simulink model "Auto_microgrid_forecasting"  (R2020a)
settings: Solver=VariableStepAuto  StartTime=0.0  StopTime=40  MaxStep=1e-4  RelTol=1e-3
PreLoadFcn:
  | %load('GC_maxRPP_WS12_GHI790_BL330_nomSOC.mat')
InitFcn:
  | run('FC_microgrid_param.m')
  | tic
  | run('CARTinitFcn.m')
StopFcn:
  | toc
undefined symbols (not defined in the file or in its folder): breakpoints1, breakpoints2, cc_kp, cp_table_data, ctrl, D1, Delta, DiscIntNeverNeededParam, DT, FC_BESS, FC_PV_FirstSolar, find_system, Fnom, forecast, GC_mode, gcbh, GHI_rated, libFC_BESS, libFC_PV, LowerLimit, magnitude, oversize, pll_ki, pll_kp, Pmax_PV, Pmax_WT, sps_rtmsupport, timer, Ts, Ts_APC, Ts_Control, Ts_Power, U_rated, UpperLimit
libraries: powerlib x146, simulink x124, powerlib_extras x120, powerlib_meascontrol x94, eePowerMeasurement x28, pi_ctrl x20, simulink_extras x12, eeGeneralControl x10, sps_avr x7, libFSArray x2, libLgBattery x1, spsDieselMotorModel x1
(part 16 of 16)

== system Auto_microgrid_forecasting/MODEL STABILIZER/AllStringInverters/Stab_control/InvControl/PLL/PLL (3ph)1/Discrete ==
  note: Use internal or external tuning parameters
  Err : Inport  SampleTime=Ts
  Constant1 : Constant  Value=Kp
  Constant3 : Constant  Value=Ki
  Discrete-Time Integrator : DiscreteIntegrator  gainval=1  InitialCondition=Init  SampleTime=Ts  LimitOutput=on  UpperSaturationLimit=Par_Limits(1)  LowerSaturationLimit=Par_Limits(2)  ICPrevOutput=DiscIntNeverNeededParam  ICPrevScaledInput=DiscIntNeverNeededParam
  Product : Product
  Product1 : Product
  Saturation1 : Saturate  UpperLimit=Par_Limits(1)  LowerLimit=Par_Limits(2)  SampleTime=Ts
  Sum6 : Sum  InputSameDT=on  SaturateOnIntegerOverflow=on  SampleTime=Ts  OutDataTypeStr=Inherit: Same as first input
  Out : Outport  SampleTime=Ts  InitialOutput=0  VectorParamsAs1DForOutWhenUnconnected=off
  wires:
  Saturation1/1 -> Out/1
  Err/1 -> Product1/1, Product/2
  Sum6/1 -> Saturation1/1
  Product/1 -> Sum6/1
  Discrete-Time Integrator/1 -> Sum6/2
  Product1/1 -> Discrete-Time Integrator/1
  Constant1/1 -> Product/1  "Kp"
  Constant3/1 -> Product1/2  "Ki"

== system Auto_microgrid_forecasting/MODEL STABILIZER/AllStringInverters/Stab_control/InvControl/PLL/PLL (3ph)1/VCO ==
  w : Inport
  Compare To Constant : simulink/Logic and Bit Operations/Compare To Constant  relop=>=  const=pi  OutDataTypeStr=uint8
  Data Type Conversion : DataTypeConversion
  Gain : Gain  Gain=2*pi  OutDataTypeStr=double
  Gain2 : Gain  Gain=Ts  SaturateOnIntegerOverflow=on  OutDataTypeStr=Inherit: Same as input  ParamDataTypeStr=Inherit: Same as input
  Sum : Sum  Inputs=-++
  Unit Delay1 : UnitDelay  SampleTime=-1  HasFrameUpgradeWarning=on
  theta : Outport  VectorParamsAs1DForOutWhenUnconnected=off
  wires:
  w/1 -> Gain2/1
  Gain/1 -> Sum/1
  Compare To Constant/1 -> Data Type Conversion/1
  Unit Delay1/1 -> Compare To Constant/1, Sum/3, theta/1  "wt"
  Gain2/1 -> Sum/2
  Sum/1 -> Unit Delay1/1
  Data Type Conversion/1 -> Gain/1

== system Auto_microgrid_forecasting/Stab1/AllStringInverters/PV_Control/InvControl/PLL/PLL (3ph)1/Discrete ==
  note: Use internal or external tuning parameters
  Err : Inport  SampleTime=Ts
  Constant1 : Constant  Value=Kp
  Constant3 : Constant  Value=Ki
  Discrete-Time Integrator : DiscreteIntegrator  gainval=1  InitialCondition=Init  SampleTime=Ts  LimitOutput=on  UpperSaturationLimit=Par_Limits(1)  LowerSaturationLimit=Par_Limits(2)  ICPrevOutput=DiscIntNeverNeededParam  ICPrevScaledInput=DiscIntNeverNeededParam
  Product : Product
  Product1 : Product
  Saturation1 : Saturate  UpperLimit=Par_Limits(1)  LowerLimit=Par_Limits(2)  SampleTime=Ts
  Sum6 : Sum  InputSameDT=on  SaturateOnIntegerOverflow=on  SampleTime=Ts  OutDataTypeStr=Inherit: Same as first input
  Out : Outport  SampleTime=Ts  InitialOutput=0  VectorParamsAs1DForOutWhenUnconnected=off
  wires:
  Constant3/1 -> Product1/2  "Ki"
  Constant1/1 -> Product/1  "Kp"
  Product1/1 -> Discrete-Time Integrator/1
  Discrete-Time Integrator/1 -> Sum6/2
  Product/1 -> Sum6/1
  Sum6/1 -> Saturation1/1
  Err/1 -> Product/2, Product1/1
  Saturation1/1 -> Out/1

== system Auto_microgrid_forecasting/Stab1/AllStringInverters/PV_Control/InvControl/PLL/PLL (3ph)1/VCO ==
  w : Inport
  Compare To Constant : simulink/Logic and Bit Operations/Compare To Constant  relop=>=  const=pi  OutDataTypeStr=uint8
  Data Type Conversion : DataTypeConversion
  Gain : Gain  Gain=2*pi  OutDataTypeStr=double
  Gain2 : Gain  Gain=Ts  SaturateOnIntegerOverflow=on  OutDataTypeStr=Inherit: Same as input  ParamDataTypeStr=Inherit: Same as input
  Sum : Sum  Inputs=-++
  Unit Delay1 : UnitDelay  SampleTime=-1  HasFrameUpgradeWarning=on
  theta : Outport  VectorParamsAs1DForOutWhenUnconnected=off
  wires:
  Data Type Conversion/1 -> Gain/1
  Sum/1 -> Unit Delay1/1
  Gain2/1 -> Sum/2
  Unit Delay1/1 -> theta/1, Sum/3, Compare To Constant/1  "wt"
  Compare To Constant/1 -> Data Type Conversion/1
  Gain/1 -> Sum/1
  w/1 -> Gain2/1

== system Auto_microgrid_forecasting/Wind Turbine Type 4/Control/Measurement and Transformation/Discrete 3-phase PLL-Driven Positive-Sequence Active & Reactive Power/Discrete 3-phase PLL-Driven Positive-Sequence Fundamental Value/Discrete Variable Frequency Mean value1/Correction subsystem ==
  N : Inport
  F : Inport  Port=2
  In : Inport  Port=3
  Gain1 : Gain  Gain=0.5  SaturateOnIntegerOverflow=on  OutDataTypeStr=Inherit: Same as input  ParamDataTypeStr=Inherit: Same as input
  Product2 : Product  Inputs=*/  InputSameDT=on  SaturateOnIntegerOverflow=on  OutDataTypeStr=Inherit: Same as first input
  Product4 : Product  Inputs=**  InputSameDT=on  SaturateOnIntegerOverflow=on  OutDataTypeStr=Inherit: Same as first input
  Product5 : Product  Inputs=**  InputSameDT=on  SaturateOnIntegerOverflow=on  OutDataTypeStr=Inherit: Same as first input
  Sum1 : Sum  Inputs=+-  InputSameDT=on  SaturateOnIntegerOverflow=on  OutDataTypeStr=Inherit: Same as first input
  Sum4 : Sum  InputSameDT=on  SaturateOnIntegerOverflow=on  OutDataTypeStr=Inherit: Same as first input
  Sum5 : Sum  Inputs=+-  InputSameDT=on  SaturateOnIntegerOverflow=on  OutDataTypeStr=Inherit: Same as first input
  Unit Delay : UnitDelay  SampleTime=Ts  HasFrameUpgradeWarning=on
  Out : Outport  VectorParamsAs1DForOutWhenUnconnected=off
  wires:
  Product4/1 -> Out/1
  Sum4/1 -> Product4/2
  Gain1/1 -> Sum4/1
  Product5/1 -> Gain1/1
  Sum1/1 -> Product5/2
  In/1 -> Sum4/2, Unit Delay/1, Sum1/1
  Product2/1 -> Product4/1
  Sum5/1 -> Product5/1, Product2/1
  F/1 -> Sum5/2
  N/1 -> Product2/2, Sum5/1
  Unit Delay/1 -> Sum1/2

== system Auto_microgrid_forecasting/Wind Turbine Type 4/Control/Measurement and Transformation/Discrete 3-phase PLL-Driven Positive-Sequence Active & Reactive Power/Discrete 3-phase PLL-Driven Positive-Sequence Fundamental Value/Discrete Variable Frequency Mean value1/Discrete Variable Transport Delay ==
  In : Inport
  D : Inport  Port=2
  "S-Function " : S-Function  FunctionName=discreteVariableTransportDelay  Parameters=MaxDelay,Ts,InitialValue  SFunctionDeploymentMode=off  EnableBusSupport=off
  Out : Outport  VectorParamsAs1DForOutWhenUnconnected=off
  wires:
  D/1 -> "S-Function "/2
  In/1 -> "S-Function "/1
  "S-Function "/1 -> Out/1

== system Auto_microgrid_forecasting/Wind Turbine Type 4/Control/Measurement and Transformation/Discrete 3-phase PLL-Driven Positive-Sequence Active & Reactive Power/Discrete 3-phase PLL-Driven Positive-Sequence Fundamental Value/Discrete Variable Frequency Mean value2/Correction subsystem ==
  N : Inport
  F : Inport  Port=2
  In : Inport  Port=3
  Gain1 : Gain  Gain=0.5  SaturateOnIntegerOverflow=on  OutDataTypeStr=Inherit: Same as input  ParamDataTypeStr=Inherit: Same as input
  Product2 : Product  Inputs=*/  InputSameDT=on  SaturateOnIntegerOverflow=on  OutDataTypeStr=Inherit: Same as first input
  Product4 : Product  Inputs=**  InputSameDT=on  SaturateOnIntegerOverflow=on  OutDataTypeStr=Inherit: Same as first input
  Product5 : Product  Inputs=**  InputSameDT=on  SaturateOnIntegerOverflow=on  OutDataTypeStr=Inherit: Same as first input
  Sum1 : Sum  Inputs=+-  InputSameDT=on  SaturateOnIntegerOverflow=on  OutDataTypeStr=Inherit: Same as first input
  Sum4 : Sum  InputSameDT=on  SaturateOnIntegerOverflow=on  OutDataTypeStr=Inherit: Same as first input
  Sum5 : Sum  Inputs=+-  InputSameDT=on  SaturateOnIntegerOverflow=on  OutDataTypeStr=Inherit: Same as first input
  Unit Delay : UnitDelay  SampleTime=Ts  HasFrameUpgradeWarning=on
  Out : Outport  VectorParamsAs1DForOutWhenUnconnected=off
  wires:
  Unit Delay/1 -> Sum1/2
  N/1 -> Sum5/1, Product2/2
  F/1 -> Sum5/2
  Sum5/1 -> Product2/1, Product5/1
  Product2/1 -> Product4/1
  In/1 -> Sum1/1, Unit Delay/1, Sum4/2
  Sum1/1 -> Product5/2
  Product5/1 -> Gain1/1
  Gain1/1 -> Sum4/1
  Sum4/1 -> Product4/2
  Product4/1 -> Out/1

== system Auto_microgrid_forecasting/Wind Turbine Type 4/Control/Measurement and Transformation/Discrete 3-phase PLL-Driven Positive-Sequence Active & Reactive Power/Discrete 3-phase PLL-Driven Positive-Sequence Fundamental Value/Discrete Variable Frequency Mean value2/Discrete Variable Transport Delay ==
  In : Inport
  D : Inport  Port=2
  "S-Function " : S-Function  FunctionName=discreteVariableTransportDelay  Parameters=MaxDelay,Ts,InitialValue  SFunctionDeploymentMode=off  EnableBusSupport=off
  Out : Outport  VectorParamsAs1DForOutWhenUnconnected=off
  wires:
  "S-Function "/1 -> Out/1
  In/1 -> "S-Function "/1
  D/1 -> "S-Function "/2

== system Auto_microgrid_forecasting/Wind Turbine Type 4/Control/Measurement and Transformation/Discrete 3-phase PLL-Driven Positive-Sequence Active & Reactive Power/Discrete 3-phase PLL-Driven Positive-Sequence Fundamental Value2/Discrete Variable Frequency Mean value1/Correction subsystem ==
  N : Inport
  F : Inport  Port=2
  In : Inport  Port=3
  Gain1 : Gain  Gain=0.5  SaturateOnIntegerOverflow=on  OutDataTypeStr=Inherit: Same as input  ParamDataTypeStr=Inherit: Same as input
  Product2 : Product  Inputs=*/  InputSameDT=on  SaturateOnIntegerOverflow=on  OutDataTypeStr=Inherit: Same as first input
  Product4 : Product  Inputs=**  InputSameDT=on  SaturateOnIntegerOverflow=on  OutDataTypeStr=Inherit: Same as first input
  Product5 : Product  Inputs=**  InputSameDT=on  SaturateOnIntegerOverflow=on  OutDataTypeStr=Inherit: Same as first input
  Sum1 : Sum  Inputs=+-  InputSameDT=on  SaturateOnIntegerOverflow=on  OutDataTypeStr=Inherit: Same as first input
  Sum4 : Sum  InputSameDT=on  SaturateOnIntegerOverflow=on  OutDataTypeStr=Inherit: Same as first input
  Sum5 : Sum  Inputs=+-  InputSameDT=on  SaturateOnIntegerOverflow=on  OutDataTypeStr=Inherit: Same as first input
  Unit Delay : UnitDelay  SampleTime=Ts  HasFrameUpgradeWarning=on
  Out : Outport  VectorParamsAs1DForOutWhenUnconnected=off
  wires:
  Unit Delay/1 -> Sum1/2
  N/1 -> Sum5/1, Product2/2
  F/1 -> Sum5/2
  Sum5/1 -> Product2/1, Product5/1
  Product2/1 -> Product4/1
  In/1 -> Sum1/1, Unit Delay/1, Sum4/2
  Sum1/1 -> Product5/2
  Product5/1 -> Gain1/1
  Gain1/1 -> Sum4/1
  Sum4/1 -> Product4/2
  Product4/1 -> Out/1

== system Auto_microgrid_forecasting/Wind Turbine Type 4/Control/Measurement and Transformation/Discrete 3-phase PLL-Driven Positive-Sequence Active & Reactive Power/Discrete 3-phase PLL-Driven Positive-Sequence Fundamental Value2/Discrete Variable Frequency Mean value1/Discrete Variable Transport Delay ==
  In : Inport
  D : Inport  Port=2
  "S-Function " : S-Function  FunctionName=discreteVariableTransportDelay  Parameters=MaxDelay,Ts,InitialValue  SFunctionDeploymentMode=off  EnableBusSupport=off
  Out : Outport  VectorParamsAs1DForOutWhenUnconnected=off
  wires:
  "S-Function "/1 -> Out/1
  In/1 -> "S-Function "/1
  D/1 -> "S-Function "/2

== system Auto_microgrid_forecasting/Wind Turbine Type 4/Control/Measurement and Transformation/Discrete 3-phase PLL-Driven Positive-Sequence Active & Reactive Power/Discrete 3-phase PLL-Driven Positive-Sequence Fundamental Value2/Discrete Variable Frequency Mean value2/Correction subsystem ==
  N : Inport
  F : Inport  Port=2
  In : Inport  Port=3
  Gain1 : Gain  Gain=0.5  SaturateOnIntegerOverflow=on  OutDataTypeStr=Inherit: Same as input  ParamDataTypeStr=Inherit: Same as input
  Product2 : Product  Inputs=*/  InputSameDT=on  SaturateOnIntegerOverflow=on  OutDataTypeStr=Inherit: Same as first input
  Product4 : Product  Inputs=**  InputSameDT=on  SaturateOnIntegerOverflow=on  OutDataTypeStr=Inherit: Same as first input
  Product5 : Product  Inputs=**  InputSameDT=on  SaturateOnIntegerOverflow=on  OutDataTypeStr=Inherit: Same as first input
  Sum1 : Sum  Inputs=+-  InputSameDT=on  SaturateOnIntegerOverflow=on  OutDataTypeStr=Inherit: Same as first input
  Sum4 : Sum  InputSameDT=on  SaturateOnIntegerOverflow=on  OutDataTypeStr=Inherit: Same as first input
  Sum5 : Sum  Inputs=+-  InputSameDT=on  SaturateOnIntegerOverflow=on  OutDataTypeStr=Inherit: Same as first input
  Unit Delay : UnitDelay  SampleTime=Ts  HasFrameUpgradeWarning=on
  Out : Outport  VectorParamsAs1DForOutWhenUnconnected=off
  wires:
  Product4/1 -> Out/1
  Sum4/1 -> Product4/2
  Gain1/1 -> Sum4/1
  Product5/1 -> Gain1/1
  Sum1/1 -> Product5/2
  In/1 -> Sum4/2, Unit Delay/1, Sum1/1
  Product2/1 -> Product4/1
  Sum5/1 -> Product5/1, Product2/1
  F/1 -> Sum5/2
  N/1 -> Product2/2, Sum5/1
  Unit Delay/1 -> Sum1/2

== system Auto_microgrid_forecasting/Wind Turbine Type 4/Control/Measurement and Transformation/Discrete 3-phase PLL-Driven Positive-Sequence Active & Reactive Power/Discrete 3-phase PLL-Driven Positive-Sequence Fundamental Value2/Discrete Variable Frequency Mean value2/Discrete Variable Transport Delay ==
  In : Inport
  D : Inport  Port=2
  "S-Function " : S-Function  FunctionName=discreteVariableTransportDelay  Parameters=MaxDelay,Ts,InitialValue  SFunctionDeploymentMode=off  EnableBusSupport=off
  Out : Outport  VectorParamsAs1DForOutWhenUnconnected=off
  wires:
  D/1 -> "S-Function "/2
  In/1 -> "S-Function "/1
  "S-Function "/1 -> Out/1

== matlab function Auto_microgrid_forecasting/Wind Turbine Type 4/APC (atomic)1/Inertial Response (to df)1/FBIC/adaptive FBIC1 ==
  data: F_de input; Delta_P output; F_dr input; Wi input; P_de output; P_dr output; Act input
function [Delta_P,P_de,P_dr] = FBIC(F_de,F_dr,Wi,Act)
%Releasible kinetic energy based method by Dr. Kang 
if Act>=0.5
    
    Wmax=1;
    Wmin=0.9;
    R0=0.05;
    K0=1/R0/(Wmax^2-Wmin^2);
    
    Ri=R0*(Wmax^2-Wmin^2)/(Wi^2-Wmin^2);
    Ki=K0*(Wi^2-Wmin^2);
    P_dr=-1/Ri*F_dr;
    P_de=-Ki*F_de;
    Delta_P=P_dr+P_de;
else
    P_dr=0;
    P_de=0;
    Delta_P=0;
end

== matlab function Auto_microgrid_forecasting/Grid Feeder Protective Relay/R25 - Sync Check v0.1/deadbus fcn ==
  data: Vbus input; y output; Vline input
% Copyright (c) 2016 Massachusetts Institute of Technology
% Permission is hereby granted, free of charge, to any person obtaining a copy of this
% software and associated documentation files (the "Software"), to deal in the Software
% without restriction, including without limitation the rights to use, copy, modify,
% merge, publish, distribute, sublicense, and/or sell copies of the Software, and to
% permit persons to whom the Software is furnished to do so, subject to the following
% conditions:
%
%
% The above copyright notice and this permission notice shall be included in
% all copies or substantial portions of the Software.
%
% THE SOFTWARE IS PROVIDED "AS IS", WITHOUT WARRANTY OF ANY KIND, EXPRESS OR IMPLIED,
% INCLUDING BUT NOT LIMITED TO THE WARRANTIES OF MERCHANTABILITY, FITNESS FOR A
% PARTICULAR PURPOSE AND NONINFRINGEMENT. IN NO EVENT SHALL THE AUTHORS OR COPYRIGHT
% HOLDERS BE LIABLE FOR ANY CLAIM, DAMAGES OR OTHER LIABILITY, WHETHER IN AN ACTION
% OF CONTRACT, TORT OR OTHERWISE, ARISING FROM, OUT OF OR IN CONNECTION WITH THE
% SOFTWARE OR THE USE OR OTHER DEALINGS IN THE SOFTWARE.
%
%
%%

function y = fcn(Vbus, Vline)
%#codegen
if isnan(Vbus)
    Vbus=0;
elseif isnan(Vline)
    Vline = 0;
end

% voltage threshold for deadbus
threshold = 0.05; % @ 5%

% bounding open-circuit voltage at 120%
a = (Vbus>(0.8)) && (Vbus<1.20) && (Vline < threshold);
b = (Vline>(0.8)) && (Vline<1.20) && (Vbus < threshold);
c = (Vline<threshold) && (Vbus < threshold);
y = a||b||c;

== matlab function Auto_microgrid_forecasting/FC_PV_FirstSolar/MPPT Controller using Perturbe & Observe technique  ==
  settings: updateMethod=DISCRETE  sampleTime=Ts_Control
  data: Param input; Enabled input; V input; I input; D output
function D  = PandO(Param, Enabled, V, I)

% MPPT controller based on the Perturb & Observe algorithm.

% D output = Reference for DC link voltage (Vdc_ref) 
%
% Enabled input = 1 to enable the MPPT controller
% V input = PV array terminal voltage (V)
% I input = PV array current (A)
%
% Param input:
Dinit = Param(1);  %Initial value for Vdc_ref
Dmax = Param(2);   %Maximum value for Vdc_ref
Dmin = Param(3);   %Minimum value for Vdc_ref
deltaD = Param(4); %Increment value used to increase/decrease Vdc_ref
%  

persistent Vold Pold Dold;

dataType = 'double';

if isempty(Vold)
    Vold=0;
    Pold=0;
    Dold=Dinit;
end
P= V*I;
dV= V - Vold;
dP= P - Pold;

if dP ~= 0 & Enabled ~=0
    if dP < 0
        if dV < 0
            D = Dold + deltaD;
        else
            D = Dold - deltaD;
        end
    else
        if dV < 0
            D = Dold - deltaD;
        else
            D = Dold + deltaD;
        end    
    end
else D=Dold;
end

if D >= Dmax | D<= Dmin
    D=Dold;
end

Dold=D;
Vold=V;
Pold=P;

== matlab function Auto_microgrid_forecasting/Wind Turbine Type 4/Fault Controller (atomic) /turbine_safety  ==
  data: ctrl input Bus: ctrlBus; data input Bus: dataBus; ctrl output; timer input Bus: timerBus; timer output; faulty parameter; dt input
 function [ctrl, timer]   = turbine_safety(ctrl, data, timer, faulty, dt)
    % Fault adaptive controller. Checks various sensor readings, and
    % responds by entering the appropriate control mode, providing the
    % appropriate torque derate, and setting the appropriate timers.
          
    % if faulted, don't change anything 
    if ctrl.mode(4)+ctrl.mode(5)+ctrl.mode(6) == 0 %if not faulted
        ctrl.RP_prev = ctrl.mode(2); %0 if ctrl.cmd =0; 1 otherwise
        fields = fieldnames(faulty); %run warning logic for all faultys
        ctrl.mode = [0,0,0,0,0,0];
        for i=1:length(fields)
            ctrl.(fields{i}).state = 0;
            checkHandle = str2func(faulty.(fields{i}).checkFun); %check for warnings/faultys
            ctrl = checkHandle(data, ctrl);
            ctrl = setMode(ctrl, faulty, fields{i}); %set mode
        end
        [ctrl, timer] = setTimers(ctrl, timer, dt); %set timers and torque derate
        ctrl.modeValue = sum(ctrl.mode.*2.^linspace(0,5,6));
    else
        if ctrl.mode(6) == 1
            fprintf('EMERGENCY STOP')
        elseif ctrl.mode(5) == 1
            fprintf('OPEN LOOP NORMAL STOP')
        elseif ctrl.mode(4) == 1
            fprintf('NORMAL STOP')
        end

%     displays for testing
%         disp('ctrl.mode:')
%         disp(ctrl.mode)
%         disp('data:')
%         disp(data)
%         disp('timer:')
%         disp(timer)
%         fprintf('data = %1.0f\n', data);
%         fprintf('ctrl.Ttarget = %1.0f\n', ctrl.Ttarget);

    end

== matlab function Auto_microgrid_forecasting/Subsystem/MATLAB Function ==
  data: grid_disconnect output; f_B2 input; V_B2 input; f_B13 input; V_B13 input; PQ_CL input; PQ_NCL input; PQ_grid input; switch_grid input; PQ_BESS input; SOC_BESS input; PQ_WT input; switch_WT input; PQ_diesel input; switch_diesel input; PQ_PV input; Pest_WT input; Pest_PV input; grid_connect output; CL_switch output; NCL_switch output; BESS_switch output; BESS_mode output; BESS_PQ_cmd output; resync output; WT_switch_req output; WT_mode output; WT_PQ_cmd output; diesel_disconnect output; diesel_connect output; PV_switch output; PV_PQ_cmd output; PV_mode output; PQ_req input; timer input; timer output; try_island input; try_GC input; flag_hiSOC input; flag_hiSOC output; forecast parameter; targetSOC output; GC_mode parameter
function [grid_disconnect, grid_connect, CL_switch, NCL_switch, BESS_switch,...
    BESS_mode, BESS_PQ_cmd, resync, WT_switch_req,...
    WT_mode, WT_PQ_cmd, diesel_disconnect, diesel_connect, PV_switch,...
    PV_PQ_cmd, PV_mode, timer, flag_hiSOC, targetSOC] = fcn(f_B2, V_B2, f_B13, V_B13, PQ_CL, PQ_NCL, PQ_grid,...
    switch_grid, PQ_BESS, SOC_BESS, PQ_WT, switch_WT, PQ_diesel,...
    switch_diesel, PQ_PV, Pest_WT, Pest_PV, PQ_req, timer, try_island, try_GC, flag_hiSOC, forecast, GC_mode)
% Naming convention: for input signals, the asset comes last in the name.
% For output signals, the output comes first in the name

xloSOC = 0.01;
loSOC = 0.10;
hiSOC = 0.95;
xhiSOC = 0.99;
nomSOC = 0.7;
targetSOC = nomSOC;
SOCbuffer = 0.05;
% DEFAULT COMMANDS
WT_switch_req = 1;
PV_switch = 1;
diesel_connect = 0;
diesel_disconnect = 0;
grid_disconnect = 0;
grid_connect = 0;
CL_switch = 1;
NCL_switch = 1;
BESS_switch = 1;
BESS_mode = 1;
BESS_PQ_cmd = [1, 0];
resync = 0;
WT_mode = [2, 1]; % wind turbine modes [P_mode, Q_mode]. P_mode:1=inertial response, 2=primary frequency response, 3=cmd track, 4=MPPT. Q_mode: 1=voltage response, 2=momentary cessation, 3=cmd track, 4=zero.
WT_PQ_cmd = [1, 0];   % should I command this to balance power?
PV_PQ_cmd = [1, 0];  % should I command this to balance power?
BESS_PQ_cmd = [1, 0];
PV_mode = 0;  
P_WT = PQ_WT(1);
Q_WT = PQ_WT(2);
P_PV = PQ_PV(1);
Q_PV = PQ_PV(2);
Pmax_WT = 618460;
Qmax_WT = 618460;
Pmax_PV = 430000;
Qmax_PV = 430000;
Pmax_BESS = 1e6;
Pmin_BESS = -Pmax_BESS;
Qmax_BESS = 1e6;
Qmin_BESS = -Qmax_BESS;
U_rated = 12;  % m/s
U_min = 6;  % m/s
GHI_rated = 1000;  %W/m2

Pmin_WT = U_min^3/U_rated^3*Pmax_WT;
PQ_L = PQ_CL + PQ_NCL;
P_L = PQ_L(1);
Q_L = PQ_L(2);

f_grid_connect = 0.5; % Hz
V_grid_connect = 0.1; % pu
f_grid_discon = 1.8; % Hz
V_grid_discon = 0.3; % pu

if try_island == 0
    timer = 0;
end

switch switch_grid
    % ISLANDED CASE
    case 0
        targetSOC = targetSOC_from_forecast(forecast, U_rated, GHI_rated, Pmax_WT, Pmax_PV, U_min, nomSOC);
        WT_mode = [2, 1];
        try_island = 0; %time until islanded
        % CHOOSE BESS MODE BASED ON SOC
        if SOC_BESS > xhiSOC || SOC_BESS < xloSOC || BESS_switch == 0  % THINK ABOUT THIS LOGIC
            BESS_mode = 0; %GFL
            if switch_diesel == 0
                diesel_connect = 1;
            else
                 if SOC_BESS > xhiSOC
                    BESS_PQ_cmd = [-1, 0];
                 elseif SOC_BESS < xloSOC
                    BESS_PQ_cmd = [1, 0];
                 end
            end
        else
            BESS_mode = 1; %GFM
        end
    % CHOOSE MICROSOURCE DISPATCH BASED ON LOAD AND RESOURCE (LATER ADD
    % FORECASTING) % I think some quantities may need to be filtered or
    % time-averaged to prevent excessive switching around threshold levels
    if BESS_switch
        if P_L > (Pest_WT+ Pest_PV + Pmax_BESS) % connect diesel if other assets can't cover load
            if switch_diesel == 0
                diesel_connect = 1;
            end
        end
        if SOC_BESS < loSOC    
            if P_L > 0.9*(Pest_WT+ Pest_PV) % min(Pest_WT, P_wind)?
                disp('hi load')
                WT_switch_req = 1;
                PV_switch = 1;
                if switch_diesel == 0
                    diesel_connect = 1;
                    disp('diesel connect')
                end
        %     elseif P_L > 0.9*(Pest_WT)  
        %         WT_switch = 1;
        %         PV_switch = 1;
            else
                WT_switch_req = 1;  
                PV_switch = 1;
            end
        else
            if SOC_BESS < targetSOC
                PV_PQ_cmd =[10*(targetSOC-SOC_BESS), PV_PQ_cmd(2)];
            else
                PV_PQ_cmd = [((P_L - P_WT)/Pmax_PV), PV_PQ_cmd(2)]; % provide difference between load and wind turbine power with PV if not in loSOC
            end
        end
        
        if SOC_BESS > hiSOC
                diesel_disconnect = 1;
                PV_switch = 0;
                WT_switch_req = 0;
                flag_hiSOC = 1;
        elseif SOC_BESS > targetSOC && flag_hiSOC == 1
                PV_switch = 0;
                WT_switch_req = 0;
        elseif SOC_BESS > 0.4
            flag_hiSOC = 0;
            if P_L < (Pest_WT + Pest_PV + Pmax_BESS) && switch_diesel == 1
                diesel_disconnect = 1;
            end        
%                 if P_L < Pest_WT
%                     PV_switch = 0;
%                     WT_switch_req = 0;
%                 elseif P_L < (Pest_WT + Pest_PV)
%                     PV_switch = 0;
%                     WT_switch_req = 1;
%                 else
%                     PV_switch = 1;
%                     WT_switch_req = 1;
%                 end
        end
    end
    if try_GC % try to connect to the utility grid 
        if abs(f_B2-60) <= f_grid_connect && abs(V_B2-1) <= V_grid_connect % connect if grid stable enough
            resync = 1;
            grid_connect = 1;
        end
    end
        
        
    
    % GRID CONNECTED CASE
    case 1
        try_GC = 0;
        CL_switch = 1;
        NCL_switch = 1;
        if switch_diesel == 1
            diesel_disconnect = 1;
        end 
        hiSOC_droop = (SOC_BESS - (hiSOC - SOCbuffer))*10;
        loSOC_droop = -((loSOC + SOCbuffer) - SOC_BESS)*10;
        switch GC_mode
            case 1 % max renewable power production
                WT_switch_req = 1;
                PV_switch = 1;
                BESS_mode = 0;
                BESS_PQ_cmd = [10*(SOC_BESS-targetSOC) , 0]; % charge battery to SOC target
                WT_mode = [4, 4]; % check that my modes are updated everywhere.
                PV_PQ_cmd = [1, 0];
%                 if f_B13 > 60
%                     if SOC_BESS > (hiSOC - SOCbuffer) % if approaching hi state of charge, BESS will discharge
%                         BESS_mode = 0;
%                         BESS_PQ_cmd = [hiSOC_droop,  BESS_PQ_cmd(2)];%[max(BESS_PQ_cmd(1), 0), BESS_PQ_cmd(2)];
%                     else % if not, provide V/f droop support
%                         BESS_mode = 1;
%                     end
%                 elseif f_B13 < 60
%                     if SOC_BESS < (loSOC + SOCbuffer) % if approaching low state of charge, BESS will charge
%                         BESS_mode = 0;
%                         BESS_PQ_cmd = [loSOC_droop,  BESS_PQ_cmd(2)];%[min(BESS_PQ_cmd(1), 0), BESS_PQ_cmd(2)];
%                     else % if not, provide V/f droop support
%                         BESS_mode = 1;
%                     end
%                 end
            case 2 %grid support with V/f droop control
                WT_switch_req = 1;
                PV_switch = 1;
                WT_mode = [2, 1];
                PV_mode = 0;
                PV_PQ_cmd = [1, 0];
                BESS_mode = 0;
                BESS_PQ_cmd = [10*(SOC_BESS-targetSOC) , 0]; % charge battery to SOC target          
%                 if f_B13 > 60
%                     if SOC_BESS > (hiSOC - SOCbuffer) % if approaching hi state of charge, BESS will discharge
%                         BESS_mode = 0;
%                         BESS_PQ_cmd = [hiSOC_droop,  BESS_PQ_cmd(2)];%[max(BESS_PQ_cmd(1), 0), BESS_PQ_cmd(2)];
%                     else % if not, provide V/f droop support
%                         BESS_mode = 1;
%                     end
%                 elseif f_B13 < 60
%                     if SOC_BESS < (loSOC + SOCbuffer) % if approaching low state of charge, BESS will charge
%                         BESS_mode = 0;
%                         BESS_PQ_cmd = [loSOC_droop,  BESS_PQ_cmd(2)];%[min(BESS_PQ_cmd(1), 0), BESS_PQ_cmd(2)];
%                     else % if not, provide V/f droop support
%                         BESS_mode = 1;
%                     end
%                 end
            case 3  % Real and reactive power tracking
                WT_switch_req = 1;
                PV_switch = 1;
                BESS_mode = 0;
                WT_mode = [3, 3];
                P_req = PQ_req(1);
                Q_req = PQ_req(2);
                Q_need = Q_req + Q_L;
                P_need = P_req + P_L;
                
                % REAL POWER PRODUCTION LOGIC
                if P_need < Pmin_WT
                    disp('P_need<Pmin_WT. PV, BESS on');
                    WT_switch_req = 0;
                    PV_switch = 1;
                    PV_PQ_cmd = [(P_need/Pmax_PV), PV_PQ_cmd(2)]; % provide as much as possible from PV
                    BESS_PQ_cmd = [((P_need - P_PV)/Pmax_BESS), BESS_PQ_cmd(2)]; % provide the rest with BESS                    
%                 elseif (Pmin_WT <= P_need) && (P_need <= Pest_WT)
%                     disp('Pmin_WT<P_need<Pest_WT. WT, BESS on')
%                     WT_switch_req = 1;
%                     PV_switch = 0;
%                     WT_PQ_cmd = [(P_need/Pmax_WT), WT_PQ_cmd(2)]; % provide as much as possible from WT                  
%                     PQ_BESS_cmd = [((P_need - P_WT)/Pmax_BESS), PQ_BESS_cmd(2)]; % provide the rest with BESS
                else  % note, combined the previous case into this one...with PV backing up WT always
                    disp('P_need>Pest_WT. WT, PV, BESS on');
                    WT_switch_req = 1;
                    PV_switch = 1;      
                    WT_PQ_cmd = [(P_need/Pmax_WT), WT_PQ_cmd(2)];
                    PV_PQ_cmd = [((P_need - P_WT)/Pmax_PV), PV_PQ_cmd(2)]; % provide as much of the rest as possible with PV
                    BESS_PQ_cmd = [((P_need - (P_WT+P_PV))/Pmax_BESS), BESS_PQ_cmd(2)]; % provide the rest with BESS
                end
                % REACTIVE POWER PRODUCTION LOGIC
                % For Q, have WT provide as much as possible, then PV, then
                % BESS. Should work regardless of what's online or not.
                WT_PQ_cmd = [WT_PQ_cmd(1), (Q_need/Qmax_WT)];
                PV_PQ_cmd = [PV_PQ_cmd(1), ((Q_need-Q_WT)/Qmax_PV)];
                if SOC_BESS > (hiSOC - SOCbuffer) % if approaching hi state of charge, BESS will discharge
                    BESS_PQ_cmd = [max(BESS_PQ_cmd(1), hiSOC_droop),  BESS_PQ_cmd(2)];
                elseif SOC_BESS < (loSOC + SOCbuffer) % if approaching low state of charge, BESSwill charge
                    BESS_PQ_cmd = [min(BESS_PQ_cmd(1), loSOC_droop),  BESS_PQ_cmd(2)];
                end
                BESS_PQ_cmd = [BESS_PQ_cmd(1), ((Q_need-Q_WT-Q_PV)/Qmax_BESS)];
                disp('Q_need')
                disp(Q_need)
                disp('Q_WT')
                disp(Q_WT)
                disp('Q_PV')
                disp(Q_PV)
                disp('Q_BESS')
                disp(PQ_BESS(2))
                disp('Q_grid')
                disp(PQ_grid(2))
%                 if WT_switch_req == 1  %can the WT just provide Q?
%                     disp('WT is on')
%                     WT_PQ_cmd = [WT_PQ_cmd(1), (Q_need/Qmax_WT)];
%                     if PV_switch == 1
%                         disp('so is PV')
%                         PV_PQ_cmd = [PV_PQ_cmd(1), ((Q_need-Q_WT)/Qmax_PV)];
%                     end
%                     BESS_PQ_cmd = [BESS_PQ_cmd(1), ((Q_need-Q_WT-Q_PV)/Qmax_BESS)];
%                 elseif PV_switch == 1
%                     disp('PV but not WT is on')
%                     PV_PQ_cmd = [PV_PQ_cmd(1), (Q_need/Qmax_PV)];
%                     BESS_PQ_cmd = [BESS_PQ_cmd(1), ((Q_need-Q_PV)/Qmax_BESS)];
%                 else
%                     BESS_PQ_cmd = [BESS_PQ_cmd(1), (Q_need/Qmax_BESS)];
%                 end  
%                 if SOC_BESS > hiSOC
%                     disp('BESS hiSOC')
%                     BESS_PQ_cmd = [max(BESS_PQ_cmd(1), 0), BESS_PQ_cmd(2)];
%                 elseif SOC_BESS < loSOC
%                     disp('BESS loSOC')
%                     BESS_PQ_cmd = [min(BESS_PQ_cmd(1), 0), BESS_PQ_cmd(2)];
%                 end
        end
        
        % ISLANDING LOGIC
        % ISLAND IF GRID UNSTABLE
        if abs(f_B2-60) > f_grid_discon || abs(V_B2-1) > V_grid_discon % disconnect if grid unstable
                BESS_mode = 1;
                grid_disconnect = 1;
        end
        % TRY TO ISLAND IF REQUESTED
        if try_island
            WT_switch_req = 1;
            PV_switch = 1;
            WT_PQ_cmd = [1, 0];
            PV_PQ_cmd = [1, 0];
            timer = timer + 0.1;
            BESS_mode = 1;
            diesel_disconnect = 0;
            if P_L > (Pmax_BESS + Pest_WT + Pest_PV)  
                disp('need diesel to island')
                diesel_connect = 1;
%                 else
%                     grid_disconnect = 1;
%             elseif P_L > (Pmax_BESS + P_WT + P_PV) 
%                 disp('need to ramp up WT, PV to island')
%                 WT_switch_req = 1;
%                 PV_switch = 1;
%                 WT_PQ_cmd = [1, 0];
%                 PV_PQ_cmd = [1, 0];
            end
            if timer > 10
                diesel_connect = 1;
            end
            if P_L < (Pmax_BESS + P_WT + P_PV) %if the local assets are providing enough power for the battery to handle the transition
                disp('enough BESS headroom to island')
                grid_disconnect = 1;
            end
        end
    end
end
%                 if f_B2 > 60
%                     if SOC_BESS > hiSOC % if hi state of charge, BESS won't absorb more P
%                         BESS_mode = 0;
%                         BESS_PQ_cmd = [0,  BESS_PQ_cmd(2)];%[max(BESS_PQ_cmd(1), 0), BESS_PQ_cmd(2)];
%                     else % if not, provide V/f droop support
%                         BESS_mode = 1;
%                     end
%                 elseif f_B2 < 60
%                     if SOC_BESS < loSOC % if lo state of charge, BESS won't inject more P
%                         BESS_mode = 0;
%                         BESS_PQ_cmd = [0,  BESS_PQ_cmd(2)];%[min(BESS_PQ_cmd(1), 0), BESS_PQ_cmd(2)];
%                     else % if not, provide V/f droop support
%                         BESS_mode = 1;
%                     end
%                 end
    
% PV_switch = 0;  % need to fix PV issue...

== matlab function Auto_microgrid_forecasting/MATLAB Function1 ==
  data: MGCC_out output; MGCC_in input Bus: MGCC_inbus
function MGCC_out = fcn(MGCC_in)




MGCC_out = 1;

== matlab function Auto_microgrid_forecasting/Wind Turbine Type 4/APC (atomic)1/Inertial Response (to df)/FBIC/adaptive FBIC1 ==
  data: F_de input; Delta_P output; F_dr input; Wi input; P_de output; P_dr output; Act input
function [Delta_P,P_de,P_dr] = FBIC(F_de,F_dr,Wi,Act)
%Releasible kinetic energy based method by Dr. Kang 
if Act>=0.5
    
    Wmax=1;
    Wmin=0.9;
    R0=0.05;
    K0=1/R0/(Wmax^2-Wmin^2);
    
    Ri=R0*(Wmax^2-Wmin^2)/(Wi^2-Wmin^2);
    Ki=K0*(Wi^2-Wmin^2);
    P_dr=-1/Ri*F_dr;
    P_de=-Ki*F_de;
    Delta_P=P_dr+P_de;
else
    P_dr=0;
    P_de=0;
    Delta_P=0;
end

== matlab function Auto_microgrid_forecasting/Wind Turbine Type 4/APC (atomic)1/Inertial Response (to df)/TLIC/adaptive TLIC ==
  data: recharge input; trecharge input; tIR input; Delta_P output; Act input; Ts_APC parameter; recharge output; trecharge output; tIR output
function [Delta_P, recharge, trecharge, tIR] = TLIC(recharge, trecharge, tIR, Act, Ts_APC)
%If frequency dips below deadband, provide max torque until rotor
%decelerates to x%. Then resume normal operation

Pmax = 1.3; %max power 1.3 pu

if recharge
    trecharge = trecharge + Ts_APC;
    Delta_P = 0;
    tIR = 0;
    if trecharge > 15
        recharge = 0;
    end
else
    trecharge = 0;
    if Act > 0.5 
        if tIR <= 3
            Delta_P = Pmax-1;
            tIR = tIR + Ts_APC;
        else
            Delta_P = 0;
            tIR = 0;
            recharge = 1;
        end
    else
        Delta_P = 0;
        tIR = 0;
    end
end

== matlab function Auto_microgrid_forecasting/Wind Turbine Type 4/Control/Speed & Pitch Control1/MATLAB Function1 ==
  data: U5s input; state output; wr input; switch_WT input; state input
function state = fcn(U5s, wr, switch_WT, state)
persistent t_startup
if isempty(t_startup)
    t_startup = 0;
end
Ts = 5e-5;
%states: 1-startup, 2-operational, 3-shutdown
if state == 1 % if in startup, move to operational once rotor accelerated and spent 10s in startup
    t_startup = t_startup + Ts;
   % print(t_startup)
    if t_startup >= 10 && wr >= 0.55
        state = 2;
        t_startup = 0;
    end
elseif state == 2 % if in operational, shutdown if below cutin or above cutout
    if U5s < 6 || U5s > 25
        state = 3;
    end
else % if in shutdown, enter startup if wind speed above cutout
    if U5s > 6
        state = 1;
        t_startup = 0 ; 
    end
end
if switch_WT == 0  % if WT disconnected, enter shutdown
    state = 3;
end
end

== matlab function Auto_microgrid_forecasting/Wind Turbine Type 4/APC (atomic)1/Inertial Response (to df)1/TLIC/adaptive TLIC ==
  data: recharge input; trecharge input; tIR input; Delta_P output; Act input; Ts_APC parameter; recharge output; trecharge output; tIR output
function [Delta_P, recharge, trecharge, tIR] = TLIC(recharge, trecharge, tIR, Act, Ts_APC)
%If frequency dips below deadband, provide max torque until rotor
%decelerates to x%. Then resume normal operation

Pmax = 1.3; %max power 1.3 pu

if recharge
    trecharge = trecharge + Ts_APC;
    Delta_P = 0;
    tIR = 0;
    if trecharge > 15
        recharge = 0;
    end
else
    trecharge = 0;
    if Act > 0.5 
        if tIR <= 3
            Delta_P = Pmax-1;
            tIR = tIR + Ts_APC;
        else
            Delta_P = 0;
            tIR = 0;
            recharge = 1;
        end
    else
        Delta_P = 0;
        tIR = 0;
    end
end

== matlab function Auto_microgrid_forecasting/Wind Turbine Type 4/Control/Speed & Pitch Control3/MATLAB Function ==
  data: U5s input; state output; wr input; state input
function state = fcn(U5s, wr, state)
persistent t_startup
if isempty(t_startup)
    t_startup = 0;
end
Ts = 5e-5;
%states: 1-startup, 2-operational, 3-shutdown
if state == 1 % if in startup, move to operational once rotor accelerated and spent 10s in startup
    t_startup = t_startup + Ts;
   % print(t_startup)
    if t_startup >= 10 && wr >= 0.55
        state = 2;
        t_startup = 0;
    end
elseif state == 2 % if in operational, shutdown if below cutin or above cutout
    if U5s < 6 || U5s > 25
        state = 3;
    end
else % if in shutdown, enter startup if wind speed above cutout
    if U5s > 6
        state = 1;
        t_startup = 0 ; 
    end
end

== matlab function Auto_microgrid_forecasting/Grid Feeder Protective Relay1/R25 - Sync Check v0.1/deadbus fcn ==
  data: Vbus input; y output; Vline input
% Copyright (c) 2016 Massachusetts Institute of Technology
% Permission is hereby granted, free of charge, to any person obtaining a copy of this
% software and associated documentation files (the "Software"), to deal in the Software
% without restriction, including without limitation the rights to use, copy, modify,
% merge, publish, distribute, sublicense, and/or sell copies of the Software, and to
% permit persons to whom the Software is furnished to do so, subject to the following
% conditions:
%
%
% The above copyright notice and this permission notice shall be included in
% all copies or substantial portions of the Software.
%
% THE SOFTWARE IS PROVIDED "AS IS", WITHOUT WARRANTY OF ANY KIND, EXPRESS OR IMPLIED,
% INCLUDING BUT NOT LIMITED TO THE WARRANTIES OF MERCHANTABILITY, FITNESS FOR A
% PARTICULAR PURPOSE AND NONINFRINGEMENT. IN NO EVENT SHALL THE AUTHORS OR COPYRIGHT
% HOLDERS BE LIABLE FOR ANY CLAIM, DAMAGES OR OTHER LIABILITY, WHETHER IN AN ACTION
% OF CONTRACT, TORT OR OTHERWISE, ARISING FROM, OUT OF OR IN CONNECTION WITH THE
% SOFTWARE OR THE USE OR OTHER DEALINGS IN THE SOFTWARE.
%
%
%%

function y = fcn(Vbus, Vline)
%#codegen
if isnan(Vbus)
    Vbus=0;
elseif isnan(Vline)
    Vline = 0;
end

% voltage threshold for deadbus
threshold = 0.05; % @ 5%

% bounding open-circuit voltage at 120%
a = (Vbus>(0.8)) && (Vbus<1.20) && (Vline < threshold);
b = (Vline>(0.8)) && (Vline<1.20) && (Vbus < threshold);
c = (Vline<threshold) && (Vbus < threshold);
y = a||b||c;
